simulink model "Copy_2_of_laod_arduino_2021"  (R2020b)
settings: Solver=FixedStepDiscrete  StartTime=0.0  StopTime=Inf  FixedStep=0.02  RelTol=1e-3  EnableMultiTasking=on
values from neighbouring files (symbols this model uses):
  attuatore_Amax = deg2rad(20)    [AVVIO_YAK_DATA.m]
  attuatore_Amin = deg2rad(-20)    [AVVIO_YAK_DATA.m]
  attuatore_Emax = deg2rad(25)    [AVVIO_YAK_DATA.m]
  attuatore_Emin = deg2rad(-25)    [AVVIO_YAK_DATA.m]
  attuatore_Rmax = deg2rad(25)    [AVVIO_YAK_DATA.m]
  attuatore_Rmin = deg2rad(-25)    [AVVIO_YAK_DATA.m]
  attuatore_Tmax = 0.4    [AVVIO_YAK_DATA.m]
  attuatore_Tmin = 0    [AVVIO_YAK_DATA.m]
  interventoA_05 = 6    [AVVIO_YAK_DATA.m]
  interventoA_1 = 2    [AVVIO_YAK_DATA.m]
  interventoE_05 = 7.5    [AVVIO_YAK_DATA.m]
  interventoE_1 = 3.2    [AVVIO_YAK_DATA.m]
  interventoT = 0.1    [AVVIO_YAK_DATA.m]
  inv_A = 1    [AVVIO_YAK_DATA.m]
  inv_comp_h = 1    [AVVIO_YAK_DATA.m]
  inv_E = 1    [AVVIO_YAK_DATA.m]
  inv_R = 1    [AVVIO_YAK_DATA.m]
  inv_T = 1    [AVVIO_YAK_DATA.m]
  K_AW_B_AP_quota = 1000    [AVVIO_YAK_DATA.m]
  K_AW_B_becc = -250    [AVVIO_YAK_DATA.m]
  K_AW_B_imb = 0    [AVVIO_YAK_DATA.m]
  K_AW_B_roll = 500    [AVVIO_YAK_DATA.m]
  K_imb_inv = -1    [AVVIO_YAK_DATA.m]
  Kd_h_app = 0.085    [AVVIO_YAK_DATA.m]
  Kd_h_flare = 0.01    [AVVIO_YAK_DATA.m]
  Ki_AP_quota_select = 0.014    [AVVIO_YAK_DATA.m]
  Ki_AP_rotta = 0.03    [AVVIO_YAK_DATA.m]
  Ki_AP_vel = 0.001    [AVVIO_YAK_DATA.m]
  Ki_becch = -0.064065    [AVVIO_YAK_DATA.m]
  Ki_h_app = 0.055    [AVVIO_YAK_DATA.m]
  Ki_h_cruise = 0.008    [AVVIO_YAK_DATA.m]
  Ki_h_flare = 0.07    [AVVIO_YAK_DATA.m]
  Ki_roll = 0.025    [AVVIO_YAK_DATA.m]
  Kp_AP_quota_hold_h = 0.15    [AVVIO_YAK_DATA.m]
  Kp_AP_quota_hold_l = 0.7    [AVVIO_YAK_DATA.m]
  Kp_AP_quota_select = 0.014    [AVVIO_YAK_DATA.m]
  Kp_AP_rotta = 0.7    [AVVIO_YAK_DATA.m]
  Kp_AP_vel = 0.02692    [AVVIO_YAK_DATA.m]
  Kp_becch = -0.1918    [AVVIO_YAK_DATA.m]
  Kp_comp_h = 0.035    [AVVIO_YAK_DATA.m]
  Kp_h_app_max = 0.086    [AVVIO_YAK_DATA.m]
  Kp_h_app_min = 0.01    [AVVIO_YAK_DATA.m]
  Kp_h_cruise = 0.04    [AVVIO_YAK_DATA.m]
  Kp_h_flare = 0.1    [AVVIO_YAK_DATA.m]
  Kp_imb = -0.04    [AVVIO_YAK_DATA.m]
  Kp_p = 0.025    [AVVIO_YAK_DATA.m]
  Kp_q = -0.025    [AVVIO_YAK_DATA.m]
  Kp_roll = 0.11    [AVVIO_YAK_DATA.m]
  Kp_Rotta_ATO = 4    [AVVIO_YAK_DATA.m]
  safe_phi = 55    [AVVIO_YAK_DATA.m]
  safe_V = 40    [AVVIO_YAK_DATA.m]
  t_AP = 0.02    [AVVIO_YAK_DATA.m]
  time_alarm_SAFE = 1    [AVVIO_YAK_DATA.m]
  V_max = 35    [AVVIO_YAK_DATA.m]
  V_stall = 15    [AVVIO_YAK_DATA.m]
  vel_wp1_al = 25    [AVVIO_YAK_DATA.m]
  vel_wp2_al = 20    [AVVIO_YAK_DATA.m]
undefined symbols (not defined in the file or in its folder): DiscIntNeverNeededParam, Newton, phi_max, phi_min, Raphson, theta_max, theta_min, tsamp
libraries: simulink_extras x43, arduinolib x26, pid_lib x8, svdutilitieslib x6, simulink x3, dspsigops x3, aerolibtransform2sys x2, aerolibtransform2 x2, cstblocks x1
(part 4 of 8)

== system Copy_2_of_laod_arduino_2021/AUTOPILOTA/Subsystem1/DECOLLO AUTOMATICO ==
  Tas : Inport
  h : Inport  Port=2
  modo : Inport  Port=3
  psi_imu : Inport  Port=4
  theta : Inport  Port=5
  V_ : Inport  Port=6
  Enable : EnablePort
  Chart1 : Stateflow chart  TreatAsAtomicUnit=on
  Memory : Memory
  Memory1 : Memory
  Radians to Degrees : simulink_extras/Transformations/Radians to Degrees
  Radians to Degrees1 : simulink_extras/Transformations/Radians to Degrees
  Sample and Hold : dspsigops/Sample and Hold  trig=Rising edge  initCond=0  latchinput=off
  Sample and Hold1 : dspsigops/Sample and Hold  trig=Rising edge  initCond=0  latchinput=off
  rotta_ATO : Outport  VectorParamsAs1DForOutWhenUnconnected=off
  Fase_ATO : Outport  Port=2  VectorParamsAs1DForOutWhenUnconnected=off
  manetta_ref_ATO : Outport  Port=3  VectorParamsAs1DForOutWhenUnconnected=off
  eq_rot_ATO : Outport  Port=4  VectorParamsAs1DForOutWhenUnconnected=off
  phi_ref_ATO : Outport  Port=5  VectorParamsAs1DForOutWhenUnconnected=off
  theta_ref_ATO : Outport  Port=6  VectorParamsAs1DForOutWhenUnconnected=off
  h_ref_ATO : Outport  Port=7  VectorParamsAs1DForOutWhenUnconnected=off
  Tas_ref_ATO : Outport  Port=8  VectorParamsAs1DForOutWhenUnconnected=off
  RC_ref_ATO : Outport  Port=9  VectorParamsAs1DForOutWhenUnconnected=off
  wires:
  Chart1/3(psi_ref) -> rotta_ATO/1  "ROTTA"
  modo/1 -> Chart1/1(modo)
  h/1 -> Chart1/3(h)
  Tas/1 -> Chart1/2(TAS)
  Chart1/10(psi_ref_selector) -> Memory/1
  Memory/1 -> Sample and Hold/Trigger
  Sample and Hold/1 -> Chart1/4(psi_hold)
  psi_imu/1 -> Radians to Degrees1/1
  Chart1/1(Fase_ATO) -> Fase_ATO/1
  Chart1/2(manetta_ref) -> manetta_ref_ATO/1
  Chart1/7(h_ref) -> h_ref_ATO/1
  Chart1/4(eq_rot) -> eq_rot_ATO/1
  Chart1/5(phi_ref) -> phi_ref_ATO/1
  Chart1/6(pitch_ref) -> theta_ref_ATO/1
  Chart1/8(Tas_ref) -> Tas_ref_ATO/1
  Chart1/9(RC_ref) -> RC_ref_ATO/1
  Sample and Hold1/1 -> Chart1/5(theta_ground_hold)
  Chart1/11(theta_ground_selector) -> Memory1/1
  Memory1/1 -> Sample and Hold1/Trigger
  theta/1 -> Radians to Degrees/1
  Radians to Degrees/1 -> Sample and Hold1/1
  V_/1 -> Chart1/6(V_)
  Radians to Degrees1/1 -> Sample and Hold/1

== system Copy_2_of_laod_arduino_2021/AUTOPILOTA/Subsystem1/Subsystem ==
  In1 : Inport
  In2 : Inport  Port=2
  In3 : Inport  Port=3
  In4 : Inport  Port=4
  In5 : Inport  Port=5
  <IAS> : Inport  Port=6
  In7 : Inport  Port=7
  <ALT> : Inport  Port=8
  <HDG> : Inport  Port=9
  In10 : Inport  Port=10
  <RC> : Inport  Port=11
  In12 : Inport  Port=12
  <Ingaggio_AP> : Inport  Port=13
  In14 : Inport  Port=14
  Enable : EnablePort
  Abs : Abs
  Data Type Conversion{,1..3} (4 alike) : DataTypeConversion  OutDataTypeStr=double
  Memory{,1..3,6} (5 alike) : Memory  InheritSampleTime=on
  Radians to Degrees3 : simulink_extras/Transformations/Radians to Degrees
  VETTORIALE : MATLAB Function  TreatAsAtomicUnit=on
  Out1 : Outport  VectorParamsAs1DForOutWhenUnconnected=off
  Out2 : Outport  Port=2  VectorParamsAs1DForOutWhenUnconnected=off
  Out3 : Outport  Port=3  VectorParamsAs1DForOutWhenUnconnected=off
  Out4 : Outport  Port=4  VectorParamsAs1DForOutWhenUnconnected=off
  wires:
  Data Type Conversion1/1 -> VETTORIALE/8(VELOCITA)
  Memory1/1 -> VETTORIALE/18(ALT_pre)
  VETTORIALE/5(ingaggio_AP_mem) -> Memory6/1
  Data Type Conversion2/1 -> VETTORIALE/9(QUOTA)
  VETTORIALE/8(ALT_pre_mem) -> Memory1/1
  Radians to Degrees3/1 -> VETTORIALE/11(HEADING)
  Memory6/1 -> VETTORIALE/15(ingaggio_AP_pre)
  In12/1 -> VETTORIALE/13(h)
  Memory3/1 -> VETTORIALE/16(modo_pre)
  VETTORIALE/6(modo_pre_mem) -> Memory3/1
  Abs/1 -> VETTORIALE/10(RC)
  VETTORIALE/9(HDG_pre_mem) -> Memory/1
  Data Type Conversion3/1 -> Abs/1
  Memory/1 -> VETTORIALE/19(HDG_pre)
  Data Type Conversion/1 -> VETTORIALE/7(ROTTA)
  Memory2/1 -> VETTORIALE/17(IAS_pre)
  VETTORIALE/7(IAS_pre_mem) -> Memory2/1
  VETTORIALE/3(rotta_vett) -> Out3/1
  In1/1 -> VETTORIALE/1(modo)
  <ALT>/1 -> VETTORIALE/3(ALT)
  <RC>/1 -> VETTORIALE/5(I_RC)
  In5/1 -> Data Type Conversion3/1
  In4/1 -> Data Type Conversion2/1
  <Ingaggio_AP>/1 -> VETTORIALE/6(ingaggio_AP)
  In10/1 -> VETTORIALE/12(TAS)
  In7/1 -> Radians to Degrees3/1
  In3/1 -> Data Type Conversion1/1
  VETTORIALE/1(V_vett) -> Out1/1
  VETTORIALE/2(h_vett) -> Out2/1
  <IAS>/1 -> VETTORIALE/2(IAS)
  In2/1 -> Data Type Conversion/1
  In14/1 -> VETTORIALE/14(RC_default)
  VETTORIALE/4(RC_vett) -> Out4/1
  <HDG>/1 -> VETTORIALE/4(HDG)

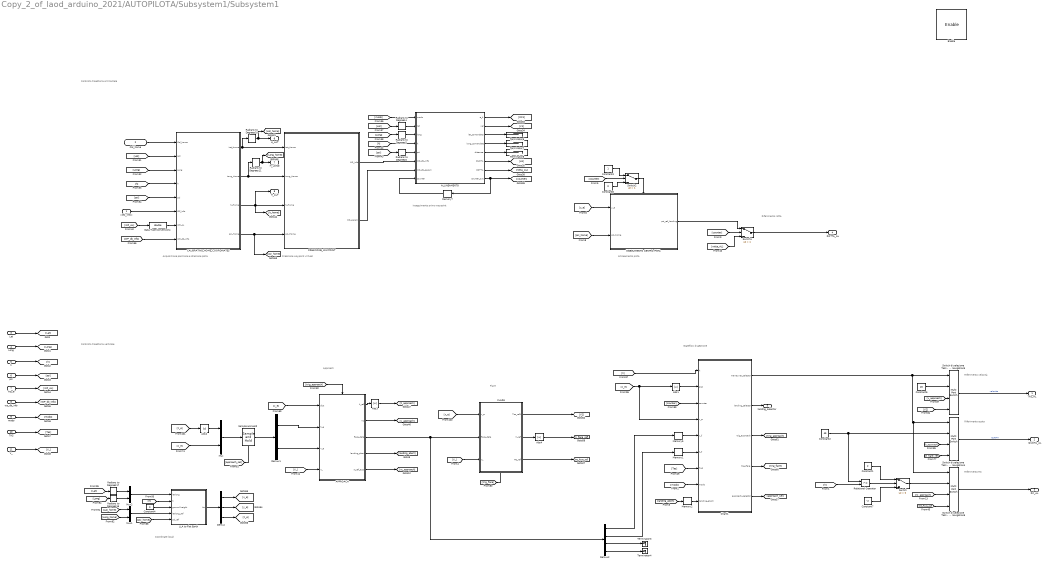
== system Copy_2_of_laod_arduino_2021/AUTOPILOTA/Subsystem1/Subsystem1 ==
  note: Approach
  note: Controllo traiettoria verticale
  note: Flare
  note: Coordinate locali
  note: Stateflow di gestione
  note: Controllo traiettoria orizzontale
  note: Acquisizione posizione
      | e direzione pista
  note: Creazione waypoint
      | virtuali
  note: Inseguimento primo
      | waypoint
  note: Allineamento
      | pista
  note: Riferimento rotta
  note: Riferimento velocità
  note: Riferimento quota
  note: Riferimento RC
  <GC_info> : Inport
  Cal_home : Inport  Port=2
  Lat : Inport  Port=3
  Long : Inport  Port=4
  h : Inport  Port=5
  psi : Inport  Port=6
  wp_al : Inport  Port=7
  wp_db_info : Inport  Port=8
  modo : Inport  Port=9
  TAS : Inport  Port=10
  V_ : Inport  Port=11
  Enable : EnablePort
  ALLINEAMENTO : MATLAB Function  TreatAsAtomicUnit=on
  APPROACH : Subsystem
  Abs{1..4} (4 alike) : Abs
  CALIBRATING_HOME_COORDINATES : MATLAB Function  TreatAsAtomicUnit=on
  "CREAZIONE_WAYPOINT " : Subsystem
  Chart1 : Stateflow chart  TreatAsAtomicUnit=on
  Constant1 : Constant  Value=2  SampleTime=0.02
  Constant2 : Constant  Value=45  SampleTime=0.02
  Constant3 : Constant
  Constant4 : Constant  Value=0  SampleTime=0.02
  Constant6 : Constant  Value=20  SampleTime=0.02
  Constant7 : Constant  Value=-2  SampleTime=0.02
  Constant8 : Constant  Value=0
  Data Type Conversion4 : DataTypeConversion  OutDataTypeStr=double
  Demux : Demux  Outputs=3
  Demux1 : Demux  Outputs=2
  Demux2 : Demux
  FLARE : Subsystem
  INSEGUIMENTO CENTRO PISTA : Subsystem
  LLA to Flat Earth : Subsystem
  Memory1 : Memory
  Memory2 : Memory
  Memory5 : Memory
  Memory7 : Memory  InitialCondition=1  InheritSampleTime=on
  Mux : Mux  Inputs=2
  Mux1 : Mux  Inputs=2
  Mux2 : Mux  Inputs=2
  Radians to Degrees{4..6,10..11,16..17} (7 alike) : simulink_extras/Transformations/Radians to Degrees
  Relational Operator : RelationalOperator  OutDataTypeStr=boolean  RndMeth=Simplest
  Sample and Hold : dspsigops/Sample and Hold  trig=Rising edge  initCond=[0 0]  latchinput=off
  Switch : Switch  Criteria=u2 > Threshold
  Switch di selezione Task - Waypoint navigation4 : MultiPortSwitch
  Switch di selezione Task - Waypoint navigation5 : MultiPortSwitch
  Switch di selezione Task - Waypoint navigation6 : MultiPortSwitch
  Switch1 : Switch  Criteria=u2 > Threshold  Threshold=1
  Switch2 : Switch  Criteria=u2 > Threshold  Threshold=1
  Terminator{3..4,6..8} (5 alike) : Terminator
  TAS_AL : Outport  VectorParamsAs1DForOutWhenUnconnected=off
  QUOTA_AL : Outport  Port=2  VectorParamsAs1DForOutWhenUnconnected=off
  RC_AL : Outport  Port=3  VectorParamsAs1DForOutWhenUnconnected=off
  ROTTA_AL : Outport  Port=4  VectorParamsAs1DForOutWhenUnconnected=off
  landing_selector : Outport  Port=5  VectorParamsAs1DForOutWhenUnconnected=off
  H_LAT : Outport  Port=6  VectorParamsAs1DForOutWhenUnconnected=off
  H_LONG : Outport  Port=7  VectorParamsAs1DForOutWhenUnconnected=off
  H_ALT : Outport  Port=8  VectorParamsAs1DForOutWhenUnconnected=off
  wires:
  Chart1/1(maneuver_selector) -> Switch di selezione Task - Waypoint navigation6/1, Switch di selezione Task - Waypoint navigation4/1, Switch di selezione Task - Waypoint navigation5/1
  LLA to Flat Earth/1(Xe) -> Demux/1
  Radians to Degrees11/1 -> H_LONG/1, [Long_home]
  Mux/1 -> Sample and Hold/1
  ALLINEAMENTO/4(long_comandato) -> Terminator7/1
  Mux1/1 -> LLA to Flat Earth/4(latlong_ref)
  [WP_db_info] -> CALIBRATING_HOME_COORDINATES/8(WP_db_info)
  Demux1/2 -> APPROACH/3(x_g)
  Abs2/1 -> Mux/1
  ALLINEAMENTO/3(lat_comandato) -> Terminator6/1
  [rc_approach] -> Switch di selezione Task - Waypoint navigation6/3
  [V2] -> Switch di selezione Task - Waypoint navigation5/4
  [x_e] -> Chart1/4(x_e), Abs1/1
  Abs4/1 -> [h_flare_ref]
  CALIBRATING_HOME_COORDINATES/3(h_Home) -> H_ALT/1, [h_home], "CREAZIONE_WAYPOINT "/3(h_Home)
  [h] -> Chart1/1(h)
  [x_e] -> FLARE/1(x_e)
  [Long_home] -> Mux1/2
  APPROACH/3(flare_data) -> Demux2/1, FLARE/2(flare_data)
  CALIBRATING_HOME_COORDINATES/1(Lat_Home) -> Radians to Degrees10/1, "CREAZIONE_WAYPOINT "/1(Lat_Home)
  Demux/2 -> [y_e]
  FLARE/3(RC_ref) -> [RC_flare_ref]
  Chart1/4(trig_flare) -> [trig_flare]
  [h] -> LLA to Flat Earth/2(h)
  [Long] -> Radians to Degrees16/1
  Demux/3 -> [z_e]
  Demux2/2 -> Memory1/1
  Radians to Degrees10/1 -> H_LAT/1, [Lat_home]
  Sample and Hold/1 -> Demux1/1
  [trig_approach] -> APPROACH/Enable
  Switch/1 -> Switch di selezione Task - Waypoint navigation6/2
  Memory5/1 -> Chart1/5(x_f)
  Cal_home/1 -> CALIBRATING_HOME_COORDINATES/1(Cal_home)
  Demux2/3 -> Terminator3/1
  FLARE/2(h_ref) -> Abs4/1
  [z_e] -> Abs2/1
  [x_e] -> Mux/2
  CALIBRATING_HOME_COORDINATES/2(Long_Home) -> "CREAZIONE_WAYPOINT "/2(Long_Home), Radians to Degrees11/1
  Demux2/4 -> Terminator4/1
  FLARE/1(Tas_ref1) -> [V2]
  ALLINEAMENTO/7(ROTTA) -> [rotta_AL]
  APPROACH/2(V1) -> [v_approach]
  [V_] -> FLARE/3(V_)
  Chart1/5(approach_selector) -> [approach_sel]
  Abs1/1 -> Chart1/2(dist)
  [h_approach] -> Switch di selezione Task - Waypoint navigation4/3
  [RC_flare_ref] -> Switch di selezione Task - Waypoint navigation6/4
  Chart1/3(trig_approach) -> [trig_approach]
  [Lat_home] -> Mux1/1
  ALLINEAMENTO/6(QUOTA) -> [H1]
  ALLINEAMENTO/8(counter_out) -> Memory7/1, [counter]
  Demux/1 -> [x_e]
  Demux2/1 -> Memory5/1
  CALIBRATING_HOME_COORDINATES/4(psi_Home) -> [psi_home], "CREAZIONE_WAYPOINT "/4(psi_Home)
  Abs3/1 -> [h_approach]
  Mux2/1 -> LLA to Flat Earth/1(latlong)
  Chart1/2(landing_selector) -> landing_selector/1
  Constant2/1 -> Switch di selezione Task - Waypoint navigation4/2, Relational Operator/1
  [h_flare_ref] -> Switch di selezione Task - Waypoint navigation4/4
  [v_approach] -> Switch di selezione Task - Waypoint navigation5/3
  [Tas] -> Chart1/7(TAS)
  APPROACH/1(h_ref) -> Abs3/1
  Data Type Conversion4/1 -> CALIBRATING_HOME_COORDINATES/7(WP_AL)
  [Lat] -> Radians to Degrees17/1
  Demux1/1 -> APPROACH/2(h_g)
  Constant4/1 -> LLA to Flat Earth/3(ground height)
  [psi] -> CALIBRATING_HOME_COORDINATES/5(psi)
  ALLINEAMENTO/2(vel) -> [V1]
  Radians to Degrees5/1 -> ALLINEAMENTO/3(long)
  [x_e] -> APPROACH/1(dist)
  Memory7/1 -> ALLINEAMENTO/8(counter)
  [h] -> CALIBRATING_HOME_COORDINATES/4(h)
  [counter] -> Chart1/3(counter)
  Radians to Degrees4/1 -> ALLINEAMENTO/2(lat)
  [approach_sel] -> Sample and Hold/Trigger
  [Lat] -> Radians to Degrees4/1
  "CREAZIONE_WAYPOINT "/2(WP_param) -> ALLINEAMENTO/7(WP_db_param)
  [h] -> ALLINEAMENTO/4(h)
  [Long] -> Radians to Degrees5/1
  <GC_info>/1 -> CALIBRATING_HOME_COORDINATES/6(GC_info)
  ALLINEAMENTO/1(e_h) -> [RC1]
  Radians to Degrees6/1 -> ALLINEAMENTO/5(psi)
  Radians to Degrees16/1 -> Mux2/2
  [psi] -> Radians to Degrees6/1
  [WP_AL] -> Data Type Conversion4/1
  [modo] -> ALLINEAMENTO/1(modo)
  ALLINEAMENTO/5(distance) -> Terminator8/1
  Radians to Degrees17/1 -> Mux2/1
  "CREAZIONE_WAYPOINT "/1(WP_info) -> ALLINEAMENTO/6(WP_db_info)
  [trig_flare] -> FLARE/Enable
  Constant6/1 -> Switch di selezione Task - Waypoint navigation5/2
  [psi_home] -> LLA to Flat Earth/5(psi_ref)
  Switch di selezione Task - Waypoint navigation4/1 -> QUOTA_AL/1  "QUOTA"
  Switch di selezione Task - Waypoint navigation6/1 -> RC_AL/1
  Switch di selezione Task - Waypoint navigation5/1 -> TAS_AL/1  "velocita"
  Lat/1 -> [Lat]
  Long/1 -> [Long]
  h/1 -> [h]
  psi/1 -> [psi]
  wp_al/1 -> [WP_AL]
  wp_db_info/1 -> [WP_db_info]
  modo/1 -> [modo]
  TAS/1 -> [Tas]
  V_/1 -> [V_]
  Switch1/1 -> ROTTA_AL/1
  [h] -> Relational Operator/2
  Relational Operator/1 -> Switch/2
  Constant1/1 -> Switch/1
  Constant7/1 -> Switch/3
  [modo] -> Chart1/8(modo)
  APPROACH/4(landing_abort) -> [landing_abort]
  Memory1/1 -> Chart1/6(h_f)
  Memory2/1 -> Chart1/9(landing_abort)
  [landing_abort] -> Memory2/1
  [Lat] -> CALIBRATING_HOME_COORDINATES/2(Lat)
  [Long] -> CALIBRATING_HOME_COORDINATES/3(Long)
  [counter] -> Switch2/2
  [rotta_AL] -> Switch1/3
  [psi_home] -> INSEGUIMENTO CENTRO PISTA/2(psi_home)
  INSEGUIMENTO CENTRO PISTA/1(psi_ref_landing) -> Switch1/1
  [y_e] -> INSEGUIMENTO CENTRO PISTA/1(y_e)
  [counter] -> Switch1/2
  Constant8/1 -> Switch2/3
  Switch2/1 -> INSEGUIMENTO CENTRO PISTA/Enable
  Constant3/1 -> Switch2/1
  [V_] -> APPROACH/4(V_)
  APPROACH/5(rc_ref_app) -> [rc_approach]

== system Copy_2_of_laod_arduino_2021/AUTOPILOTA/Subsystem1/Subsystem2 ==
  In1 : Inport
  In2 : Inport  Port=2
  In3 : Inport  Port=3
  In4 : Inport  Port=4
  In5 : Inport  Port=5
  In6 : Inport  Port=6
  <GC_info> : Inport  Port=7
  Enable : EnablePort
  Memory4 : Memory  InitialCondition=1  InheritSampleTime=on
  Radians to Degrees : simulink_extras/Transformations/Radians to Degrees
  Radians to Degrees1 : simulink_extras/Transformations/Radians to Degrees
  Radians to Degrees2 : simulink_extras/Transformations/Radians to Degrees
  Terminator : Terminator
  Terminator1 : Terminator
  Terminator2 : Terminator
  WAYPOINTS : MATLAB Function  TreatAsAtomicUnit=on
  saturatore V : Saturate  UpperLimit=40  LowerLimit=15
  saturatore V1 : Saturate  UpperLimit=2  LowerLimit=-2
  RC : Outport  VectorParamsAs1DForOutWhenUnconnected=off
  VELOCITA : Outport  Port=2  VectorParamsAs1DForOutWhenUnconnected=off
  Out3 : Outport  Port=3  VectorParamsAs1DForOutWhenUnconnected=off
  Out4 : Outport  Port=4  VectorParamsAs1DForOutWhenUnconnected=off
  wires:
  WAYPOINTS/8(counter_out) -> Memory4/1
  saturatore V1/1 -> RC/1  "RC"
  Radians to Degrees1/1 -> WAYPOINTS/2(long)
  WAYPOINTS/4(long_comandato) -> Terminator1/1
  Radians to Degrees/1 -> WAYPOINTS/1(lat)
  WAYPOINTS/2(vel) -> saturatore V/1
  WAYPOINTS/1(e_h) -> saturatore V1/1
  WAYPOINTS/5(distance) -> Terminator2/1
  WAYPOINTS/3(lat_comandato) -> Terminator/1
  Radians to Degrees2/1 -> WAYPOINTS/4(psi)
  Memory4/1 -> WAYPOINTS/8(counter)
  In1/1 -> Radians to Degrees/1
  In3/1 -> WAYPOINTS/3(h)
  In4/1 -> Radians to Degrees2/1
  In2/1 -> Radians to Degrees1/1
  WAYPOINTS/7(ROTTA) -> Out4/1
  In5/1 -> WAYPOINTS/5(WP_db_info)
  In6/1 -> WAYPOINTS/6(WP_db_param)
  <GC_info>/1 -> WAYPOINTS/7(GC_info)
  saturatore V/1 -> VELOCITA/1  "VELOCITA"
  WAYPOINTS/6(QUOTA) -> Out3/1

== system Copy_2_of_laod_arduino_2021/AUTOPILOTA/Subsystem1/Subsystem3 ==
  In1 : Inport
  In2 : Inport  Port=2
  In3 : Inport  Port=3
  In4 : Inport  Port=4
  In5 : Inport  Port=5
  In6 : Inport  Port=6
  In7 : Inport  Port=7
  In8 : Inport  Port=8
  Enable : EnablePort
  GO_HOME : MATLAB Function  TreatAsAtomicUnit=on
  Radians to Degrees12 : simulink_extras/Transformations/Radians to Degrees
  Radians to Degrees13 : simulink_extras/Transformations/Radians to Degrees
  Radians to Degrees9 : simulink_extras/Transformations/Radians to Degrees
  Out1 : Outport  VectorParamsAs1DForOutWhenUnconnected=off
  Out2 : Outport  Port=2  VectorParamsAs1DForOutWhenUnconnected=off
  Out3 : Outport  Port=3  VectorParamsAs1DForOutWhenUnconnected=off
  Out4 : Outport  Port=4  VectorParamsAs1DForOutWhenUnconnected=off
  wires:
  GO_HOME/1(V_goHome) -> Out1/1
  GO_HOME/4(rotta_goHome) -> Out4/1
  GO_HOME/3(RC_goHome) -> Out3/1
  Radians to Degrees9/1 -> GO_HOME/4(psi)
  Radians to Degrees12/1 -> GO_HOME/1(lat)
  In2/1 -> Radians to Degrees13/1
  Radians to Degrees13/1 -> GO_HOME/2(long)
  In3/1 -> GO_HOME/3(h)
  In4/1 -> Radians to Degrees9/1
  In6/1 -> GO_HOME/6(Long_Home)
  In8/1 -> GO_HOME/8(V_goHome_rif)
  In5/1 -> GO_HOME/5(Lat_Home)
  In1/1 -> Radians to Degrees12/1
  GO_HOME/2(h_goHome) -> Out2/1
  In7/1 -> GO_HOME/7(h_goHome_rif)

== system Copy_2_of_laod_arduino_2021/MISURE DA SENSORI FILTRATE/TX & RX Seriale Arduino Raspberry/Subsystem1 ==
  In1 : Inport
  Enable : EnablePort
  MATLAB Function : MATLAB Function  TreatAsAtomicUnit=on
  MATLAB Function1 : MATLAB Function  Commented=on  TreatAsAtomicUnit=on
  Subsystem1 : Subsystem  Commented=on
  Subsystem2 : Subsystem
  Terminator : Terminator  Commented=on
  Transpose : Math  Operator=transpose  SignedPower=on  SaturateOnIntegerOverflow=on
  Unit Delay : UnitDelay  Commented=on  SampleTime=-1  HasFrameUpgradeWarning=on
  Single : Outport  VectorParamsAs1DForOutWhenUnconnected=off
  Int16 : Outport  Port=2  VectorParamsAs1DForOutWhenUnconnected=off
  uint16 : Outport  Port=3  VectorParamsAs1DForOutWhenUnconnected=off
  wires:
  In1/1 -> Transpose/1
  Subsystem2/1(Out2) -> Single/1
  Subsystem2/2(Out3) -> Int16/1
  Subsystem2/3(Out4) -> uint16/1
  MATLAB Function/1(status) -> Subsystem2/Enable
  MATLAB Function/2(messaggio) -> Subsystem2/1(In1)
  MATLAB Function1/1(status) -> Subsystem1/Enable
  MATLAB Function1/3(messaggio) -> Subsystem1/1(In1), Unit Delay/1
  Unit Delay/1 -> MATLAB Function1/2(mess_prec)
  MATLAB Function1/2(check) -> Terminator/1
  Transpose/1 -> MATLAB Function/1(byte_pack)

== system Copy_2_of_laod_arduino_2021/Misure Sensori/ATTOPILOT/Scalatura_bit_to_percent_Volt ==
  Bit : Inport
  Sum : Sum  Inputs=|++
  m_attopilota_bit_to_percent : Gain  Gain=100/361  ParamDataTypeStr=double
  q_attopilota_bit_to_percent : Constant  Value=-204800/361
  Percent_Volt : Outport  VectorParamsAs1DForOutWhenUnconnected=off
  wires:
  Bit/1 -> m_attopilota_bit_to_percent/1
  Sum/1 -> Percent_Volt/1
  q_attopilota_bit_to_percent/1 -> Sum/2
  m_attopilota_bit_to_percent/1 -> Sum/1

== system Copy_2_of_laod_arduino_2021/Misure Sensori/BMP_280/Dynamic rate limiter ==
  note: U(k)
  note: Y(k)
  up : Inport
  u : Inport  Port=2
  lo : Inport  Port=3
  Delay Input2 : UnitDelay  Description=Store in Global RAM  DisableCoverage=on  InitialCondition=101325  SampleTime=-1  HasFrameUpgradeWarning=on
  Difference Inputs1 : Sum  Description=Add in CPU  DisableCoverage=on  Inputs=+-  OutDataTypeStr=Inherit: Inherit via back propagation
  Difference Inputs2 : Sum  Description=Add in CPU  OutDataTypeStr=Inherit: Inherit via back propagation
  FixPt Data Type Duplicate : DataTypeDuplicate  DisableCoverage=on  NumInputPorts=7
  Saturation Dynamic : simulink/Discontinuities/Saturation Dynamic  OutMin=[]  OutMax=[]  OutDataTypeStr=Inherit: Same as second input  OutDataType=fixdt(1, 16)  OutScaling=2^-10  DoSatur=off
  delta fall limit : Product  DisableCoverage=on  Inputs=**  OutDataTypeStr=Inherit: Inherit via back propagation  SaturateOnIntegerOverflow=on
  delta rise limit : Product  DisableCoverage=on  Inputs=**  OutDataTypeStr=Inherit: Inherit via back propagation  SaturateOnIntegerOverflow=on
  sample time : SampleTimeMath  DisableCoverage=on  TsampMathOp=Ts Only  weightValue=1
  Y : Outport  InitialOutput=0  VectorParamsAs1DForOutWhenUnconnected=off
  wires:
  delta rise limit/1 -> FixPt Data Type Duplicate/6, Saturation Dynamic/1
  Difference Inputs2/1 -> Y/1, Delay Input2/1, FixPt Data Type Duplicate/1
  up/1 -> delta rise limit/1
  Saturation Dynamic/1 -> Difference Inputs2/1, FixPt Data Type Duplicate/7
  Delay Input2/1 -> Difference Inputs1/2, FixPt Data Type Duplicate/2, Difference Inputs2/2  "Y(k-1)"
  Difference Inputs1/1 -> FixPt Data Type Duplicate/4, Saturation Dynamic/2  "( U(k) - Y(k-1) )"
  u/1 -> Difference Inputs1/1, FixPt Data Type Duplicate/5, sample time/1
  lo/1 -> delta fall limit/1
  sample time/1 -> delta fall limit/2, delta rise limit/2
  delta fall limit/1 -> FixPt Data Type Duplicate/3, Saturation Dynamic/3

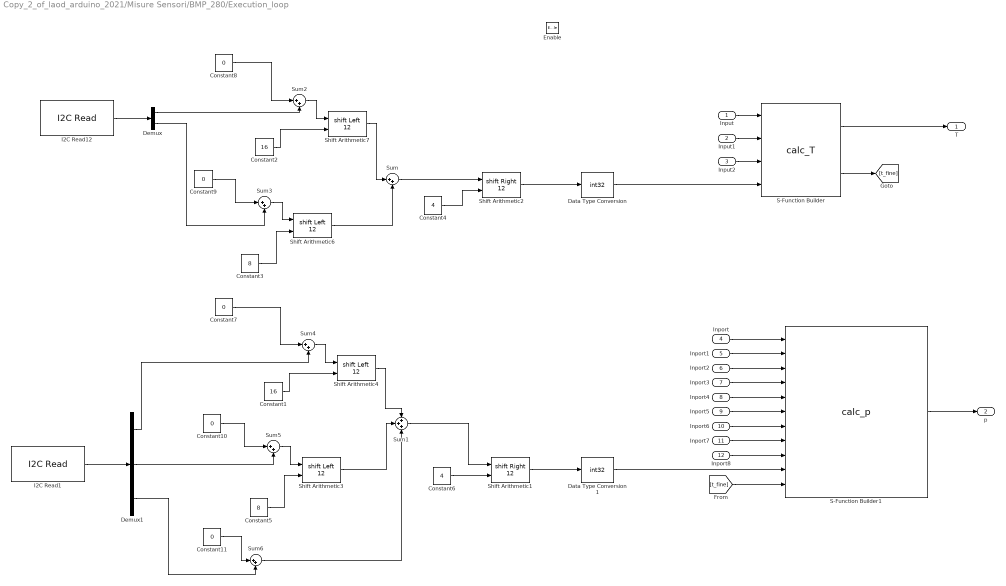
== system Copy_2_of_laod_arduino_2021/Misure Sensori/BMP_280/Execution_loop ==
  Input : Inport
  Input1 : Inport  Port=2
  Input2 : Inport  Port=3
  Inport : Inport  Port=4
  Inport1 : Inport  Port=5
  Inport2 : Inport  Port=6
  Inport3 : Inport  Port=7
  Inport4 : Inport  Port=8
  Inport5 : Inport  Port=9
  Inport6 : Inport  Port=10
  Inport7 : Inport  Port=11
  Inport8 : Inport  Port=12
  Enable : EnablePort
  Constant1 : Constant  Value=16
  Constant{7..11} (5 alike) : Constant  Value=0  OutDataTypeStr=uint32
  Constant2 : Constant  Value=16
  Constant3 : Constant  Value=8
  Constant4 : Constant  Value=4
  Constant5 : Constant  Value=8
  Constant6 : Constant  Value=4
  Data Type Conversion : DataTypeConversion  OutDataTypeStr=int32
  Data Type Conversion1 : DataTypeConversion  OutDataTypeStr=int32
  Demux : Demux  Outputs=2
  Demux1 : Demux  Outputs=3
  I2C Read1 : arduinolib/I2C Read  Priority=2  I2CModule=0  Mode=Master  SlaveAddress=hex2dec( '76' )  SlaveByteOrder=BigEndian  Direction=Receiver  RegisterAddressMode=on  RegisterAddress=hex2dec( 'F7' )  SlaveDataType=uint8  DataLength=3  NoAck=off  RepeatedStart=off  OutputStatus=off  blockPlatform=arduino  SampleTime=t_AP
      settings: AttributesFormatString=Priority=%<Priority>  SourceProductBaseCode=ARDUINO
  I2C Read12 : arduinolib/I2C Read  Priority=1  I2CModule=0  Mode=Master  SlaveAddress=hex2dec( '76' )  SlaveByteOrder=BigEndian  Direction=Receiver  RegisterAddressMode=on  RegisterAddress=hex2dec( 'FA' )  SlaveDataType=uint8  DataLength=2  NoAck=off  RepeatedStart=off  OutputStatus=off  blockPlatform=arduino  SampleTime=t_AP
      settings: AttributesFormatString=Priority=%<Priority>  SourceProductBaseCode=ARDUINO
  S-Function Builder : S-Function  InitFcn=try, set_param(gcb,'FunctionName','calc_T'), end  FunctionName=calc_T  SFunctionModules=calc_T_wrapper  SFunctionDeploymentMode=off  EnableBusSupport=off  mask(S-Function Builder){}
      mask help: Simulink:masks:SFunctionBuilder_MD
      mask init: same as Copy_2_of_laod_arduino_2021/AIR RX/S-Function Builder
      settings: CopyFcn=set_param(gcbh,'LinkStatus','none')  PreSaveFcn=try, set_param(gcb,'FunctionName','calc_T'), end  OpenFcn=sfunctionwizard(gcbh)
      mask Display: plot(val(:,1),val(:,2)),disp(sys), port_label('input',1,'dig_T1'), port_label('input',2,'dig_T2'), port_label('input',3,'dig_T3'), port_label('input',4,'adc_T'), port_label('output',1,'T'), port_label('output',2,'t_fine')
  S-Function Builder1 : S-Function  InitFcn=try, set_param(gcb,'FunctionName','calc_p'), end  FunctionName=calc_p  SFunctionModules=calc_p_wrapper  SFunctionDeploymentMode=off  EnableBusSupport=off  mask(S-Function Builder){}
      mask help: Simulink:masks:SFunctionBuilder_MD
      mask init: same as Copy_2_of_laod_arduino_2021/AIR RX/S-Function Builder
      settings: CopyFcn=set_param(gcbh,'LinkStatus','none')  PreSaveFcn=try, set_param(gcb,'FunctionName','calc_p'), end  OpenFcn=sfunctionwizard(gcbh)
      mask Display: plot(val(:,1),val(:,2)),disp(sys), port_label('input',1,'dig_p1'), port_label('input',2,'dig_p2'), port_label('input',3,'dig_p3'), port_label('input',4,'dig_p4'), port_label('input',5,'dig_p5'), port_label('input',6,'dig_p6'), port_label('input',7,'dig_p7'), port_label('input',8,'dig_p8'), port_label('input',9,'dig_p9'), port_label('input',10,'adc_P'), port_label('input',11,'t_fine'), port_label('output',1,'p')
  Shift Arithmetic1 : ArithShift  BitShiftNumberSource=Input port  BitShiftNumber=12  BitShiftDirection=Right
      settings: InputPortMap=u0,p1
  Shift Arithmetic2 : ArithShift  BitShiftNumberSource=Input port  BitShiftNumber=12  BitShiftDirection=Right
      settings: InputPortMap=u0,p1
  Shift Arithmetic{3..4,6..7} (4 alike) : ArithShift  BitShiftNumberSource=Input port  BitShiftNumber=12  BitShiftDirection=Left
      settings: InputPortMap=u0,p1
  Sum{,2..6} (6 alike) : Sum  Inputs=|++
  Sum1 : Sum  Inputs=+++
  T : Outport  VectorParamsAs1DForOutWhenUnconnected=off
  p : Outport  Port=2  VectorParamsAs1DForOutWhenUnconnected=off
  wires:
  Shift Arithmetic2/1 -> Data Type Conversion/1
  Constant4/1 -> Shift Arithmetic2/2
  S-Function Builder/1 -> T/1
  Input2/1 -> S-Function Builder/3
  Input1/1 -> S-Function Builder/2
  Input/1 -> S-Function Builder/1
  Constant3/1 -> Shift Arithmetic6/2
  Constant2/1 -> Shift Arithmetic7/2
  Shift Arithmetic7/1 -> Sum/1
  Shift Arithmetic6/1 -> Sum/2
  Sum/1 -> Shift Arithmetic2/1
  Sum2/1 -> Shift Arithmetic7/1
  Constant8/1 -> Sum2/1
  Constant9/1 -> Sum3/1
  Demux/2 -> Sum3/2
  Sum3/1 -> Shift Arithmetic6/1
  Data Type Conversion/1 -> S-Function Builder/4
  Shift Arithmetic4/1 -> Sum1/1
  Constant5/1 -> Shift Arithmetic3/2
  Shift Arithmetic1/1 -> Data Type Conversion1/1
  Constant1/1 -> Shift Arithmetic4/2
  Constant6/1 -> Shift Arithmetic1/2
  Sum1/1 -> Shift Arithmetic1/1
  Constant7/1 -> Sum4/1
  S-Function Builder1/1 -> p/1
  Sum5/1 -> Shift Arithmetic3/1
  Constant10/1 -> Sum5/1
  Demux1/2 -> Sum5/2
  Shift Arithmetic3/1 -> Sum1/2
  Sum4/1 -> Shift Arithmetic4/1
  Constant11/1 -> Sum6/1
  Demux1/3 -> Sum6/2
  Sum6/1 -> Sum1/3
  Data Type Conversion1/1 -> S-Function Builder1/10
  Inport/1 -> S-Function Builder1/1
  Inport1/1 -> S-Function Builder1/2
  Inport2/1 -> S-Function Builder1/3
  Inport3/1 -> S-Function Builder1/4
  Inport4/1 -> S-Function Builder1/5
  Inport5/1 -> S-Function Builder1/6
  Inport6/1 -> S-Function Builder1/7
  Inport7/1 -> S-Function Builder1/8
  Inport8/1 -> S-Function Builder1/9
  S-Function Builder/2 -> [t_fine]
  [t_fine] -> S-Function Builder1/11
  I2C Read12/1 -> Demux/1
  Demux/1 -> Sum2/2
  I2C Read1/1 -> Demux1/1
  Demux1/1 -> Sum4/2

== system Copy_2_of_laod_arduino_2021/Misure Sensori/BMP_280/One_time_initialization ==
  Enable : EnablePort
  Bitwise Operator1 : simulink/Logic and Bit Operations/Bitwise Operator  logicop=AND  UseBitMask=on  BitMask=hex2dec('FF')  BitMaskRealWorld=Stored Integer
  Byte Unpack : svdutilitieslib/Byte Unpack  dimensions={[8]}  datatypes={'uint16'}  byteAlign=1  blockPlatform=arduinoert
      settings: SourceProductBaseCode=ANDROID,ARDUINO,ML_ARDUINO,ECCORTEXA,ECCORTEXR,SC_BEAGLEBONE_BLUE,EC_FREEDOM_BOARD,EC_FRDM_K64F,INTEL_BLOCKSET,JETSONCPU,MICROBIT,NUCLEO,NVIDIA,PX4AUTOPILOTS,RASPPIIO,STMICRODIS,TIC2000,XILINX_BLOCKSET
  Constant1 : Constant  Value=hex2dec('0')  OutDataTypeStr=uint8  SampleTime=-1
  Constant4 : Constant  Value=hex2dec('2F')  OutDataTypeStr=uint8  SampleTime=-1
  Data Type Conversion10 : DataTypeConversion  OutDataTypeStr=uint8
  Data Type Conversion11 : DataTypeConversion  OutDataTypeStr=uint8
  I2C Read : arduinolib/I2C Read  Priority=1  I2CModule=0  Mode=Master  SlaveAddress=hex2dec( '76' )  SlaveByteOrder=LittleEndian  Direction=Receiver  RegisterAddressMode=on  RegisterAddress=hex2dec( '88' )  SlaveDataType=uint16  DataLength=1  NoAck=off  RepeatedStart=off  OutputStatus=off  blockPlatform=arduino  SampleTime=t_AP
      settings: AttributesFormatString=Priority=%<Priority>  SourceProductBaseCode=ARDUINO
  I2C Read1 : arduinolib/I2C Read  Priority=2  I2CModule=0  Mode=Master  SlaveAddress=hex2dec( '76' )  SlaveByteOrder=LittleEndian  Direction=Receiver  RegisterAddressMode=on  RegisterAddress=hex2dec( '8A' )  SlaveDataType=int16  DataLength=1  NoAck=off  RepeatedStart=off  OutputStatus=off  blockPlatform=arduino  SampleTime=t_AP
      settings: AttributesFormatString=Priority=%<Priority>  SourceProductBaseCode=ARDUINO
  I2C Read10 : arduinolib/I2C Read  Priority=11  I2CModule=0  Mode=Master  SlaveAddress=hex2dec( '76' )  SlaveByteOrder=LittleEndian  Direction=Receiver  RegisterAddressMode=on  RegisterAddress=hex2dec( '9C' )  SlaveDataType=int16  DataLength=1  NoAck=off  RepeatedStart=off  OutputStatus=off  blockPlatform=arduino  SampleTime=t_AP
      settings: AttributesFormatString=Priority=%<Priority>  SourceProductBaseCode=ARDUINO
  I2C Read11 : arduinolib/I2C Read  Priority=12  I2CModule=0  Mode=Master  SlaveAddress=hex2dec( '76' )  SlaveByteOrder=LittleEndian  Direction=Receiver  RegisterAddressMode=on  RegisterAddress=hex2dec( '9E' )  SlaveDataType=int16  DataLength=1  NoAck=off  RepeatedStart=off  OutputStatus=off  blockPlatform=arduino  SampleTime=t_AP
      settings: AttributesFormatString=Priority=%<Priority>  SourceProductBaseCode=ARDUINO
  I2C Read12 : arduinolib/I2C Read  Priority=16  I2CModule=0  Mode=Master  SlaveAddress=hex2dec( '50' )  SlaveByteOrder=BigEndian  Direction=Receiver  RegisterAddressMode=off  RegisterAddress=0  SlaveDataType=uint8  DataLength=16  NoAck=off  RepeatedStart=off  OutputStatus=off  blockPlatform=ARDUINO  SampleTime=0.02
      settings: AttributesFormatString=Priority=%<Priority>  SourceProductBaseCode=ARDUINO
  I2C Read2 : arduinolib/I2C Read  Priority=3  I2CModule=0  Mode=Master  SlaveAddress=hex2dec( '76' )  SlaveByteOrder=LittleEndian  Direction=Receiver  RegisterAddressMode=on  RegisterAddress=hex2dec( '8C' )  SlaveDataType=int16  DataLength=1  NoAck=off  RepeatedStart=off  OutputStatus=off  blockPlatform=arduino  SampleTime=t_AP
      settings: AttributesFormatString=Priority=%<Priority>  SourceProductBaseCode=ARDUINO
  I2C Read3 : arduinolib/I2C Read  Priority=4  I2CModule=0  Mode=Master  SlaveAddress=hex2dec( '76' )  SlaveByteOrder=LittleEndian  Direction=Receiver  RegisterAddressMode=on  RegisterAddress=hex2dec( '8E' )  SlaveDataType=uint16  DataLength=1  NoAck=off  RepeatedStart=off  OutputStatus=off  blockPlatform=arduino  SampleTime=t_AP
      settings: AttributesFormatString=Priority=%<Priority>  SourceProductBaseCode=ARDUINO
  I2C Read4 : arduinolib/I2C Read  Priority=5  I2CModule=0  Mode=Master  SlaveAddress=hex2dec( '76' )  SlaveByteOrder=LittleEndian  Direction=Receiver  RegisterAddressMode=on  RegisterAddress=hex2dec( '90' )  SlaveDataType=int16  DataLength=1  NoAck=off  RepeatedStart=off  OutputStatus=off  blockPlatform=arduino  SampleTime=t_AP
      settings: AttributesFormatString=Priority=%<Priority>  SourceProductBaseCode=ARDUINO
  I2C Read5 : arduinolib/I2C Read  Priority=6  I2CModule=0  Mode=Master  SlaveAddress=hex2dec( '76' )  SlaveByteOrder=LittleEndian  Direction=Receiver  RegisterAddressMode=on  RegisterAddress=hex2dec( '92' )  SlaveDataType=int16  DataLength=1  NoAck=off  RepeatedStart=off  OutputStatus=off  blockPlatform=arduino  SampleTime=t_AP
      settings: AttributesFormatString=Priority=%<Priority>  SourceProductBaseCode=ARDUINO
  I2C Read6 : arduinolib/I2C Read  Priority=7  I2CModule=0  Mode=Master  SlaveAddress=hex2dec( '76' )  SlaveByteOrder=LittleEndian  Direction=Receiver  RegisterAddressMode=on  RegisterAddress=hex2dec( '94' )  SlaveDataType=int16  DataLength=1  NoAck=off  RepeatedStart=off  OutputStatus=off  blockPlatform=arduino  SampleTime=t_AP
      settings: AttributesFormatString=Priority=%<Priority>  SourceProductBaseCode=ARDUINO
  I2C Read7 : arduinolib/I2C Read  Priority=8  I2CModule=0  Mode=Master  SlaveAddress=hex2dec( '76' )  SlaveByteOrder=LittleEndian  Direction=Receiver  RegisterAddressMode=on  RegisterAddress=hex2dec( '96' )  SlaveDataType=int16  DataLength=1  NoAck=off  RepeatedStart=off  OutputStatus=off  blockPlatform=arduino  SampleTime=t_AP
      settings: AttributesFormatString=Priority=%<Priority>  SourceProductBaseCode=ARDUINO
  I2C Read8 : arduinolib/I2C Read  Priority=9  I2CModule=0  Mode=Master  SlaveAddress=hex2dec( '76' )  SlaveByteOrder=LittleEndian  Direction=Receiver  RegisterAddressMode=on  RegisterAddress=hex2dec( '98' )  SlaveDataType=int16  DataLength=1  NoAck=off  RepeatedStart=off  OutputStatus=off  blockPlatform=arduino  SampleTime=t_AP
      settings: AttributesFormatString=Priority=%<Priority>  SourceProductBaseCode=ARDUINO
  I2C Read9 : arduinolib/I2C Read  Priority=10  I2CModule=0  Mode=Master  SlaveAddress=hex2dec( '76' )  SlaveByteOrder=LittleEndian  Direction=Receiver  RegisterAddressMode=on  RegisterAddress=hex2dec( '9A' )  SlaveDataType=int16  DataLength=1  NoAck=off  RepeatedStart=off  OutputStatus=off  blockPlatform=arduino  SampleTime=t_AP
      settings: AttributesFormatString=Priority=%<Priority>  SourceProductBaseCode=ARDUINO
  I2C Write1 : arduinolib/I2C Write  Priority=13  I2CModule=0  Mode=Master  SlaveAddress=hex2dec( '76' )  SlaveByteOrder=LittleEndian  Direction=Transmitter  RegisterAddressMode=on  RegisterAddress=hex2dec( 'F4' )  SlaveDataType=uint8  DataLength=1  NoAck=off  RepeatedStart=off  OutputStatus=off  blockPlatform=arduino
      settings: AttributesFormatString=Priority=%<Priority>  SourceProductBaseCode=ARDUINO
  I2C Write2 : arduinolib/I2C Write  Priority=14  I2CModule=0  Mode=Master  SlaveAddress=hex2dec( '76' )  SlaveByteOrder=LittleEndian  Direction=Transmitter  RegisterAddressMode=on  RegisterAddress=hex2dec( 'F5' )  SlaveDataType=uint8  DataLength=1  NoAck=off  RepeatedStart=off  OutputStatus=off  blockPlatform=arduino
      settings: AttributesFormatString=Priority=%<Priority>  SourceProductBaseCode=ARDUINO
  I2C Write3 : arduinolib/I2C Write  Priority=15  I2CModule=0  Mode=Master  SlaveAddress=hex2dec( '50' )  SlaveByteOrder=BigEndian  Direction=Transmitter  RegisterAddressMode=off  RegisterAddress=hex2dec( '0' )  SlaveDataType=uint8  DataLength=1  NoAck=off  RepeatedStart=off  OutputStatus=off  blockPlatform=ARDUINO
      settings: AttributesFormatString=Priority=%<Priority>  SourceProductBaseCode=ARDUINO
  Mux1 : Mux  Inputs=2
  Shift Arithmetic1 : ArithShift  BitShiftNumber=8  BitShiftDirection=Right
  "registro memoria2 " : Constant  Value=0  OutDataTypeStr=uint16  SampleTime=t_AP
  dig_T1 : Outport  VectorParamsAs1DForOutWhenUnconnected=off
  dig_T2 : Outport  Port=2  VectorParamsAs1DForOutWhenUnconnected=off
  dig_T3 : Outport  Port=3  VectorParamsAs1DForOutWhenUnconnected=off
  dig_p1 : Outport  Port=4  VectorParamsAs1DForOutWhenUnconnected=off
  dig_p2 : Outport  Port=5  VectorParamsAs1DForOutWhenUnconnected=off
  dig_p3 : Outport  Port=6  VectorParamsAs1DForOutWhenUnconnected=off
  dig_p4 : Outport  Port=7  VectorParamsAs1DForOutWhenUnconnected=off
  dig_p5 : Outport  Port=8  VectorParamsAs1DForOutWhenUnconnected=off
  dig_p6 : Outport  Port=9  VectorParamsAs1DForOutWhenUnconnected=off
  dig_p7 : Outport  Port=10  VectorParamsAs1DForOutWhenUnconnected=off
  dig_p8 : Outport  Port=11  VectorParamsAs1DForOutWhenUnconnected=off
  dig_p9 : Outport  Port=12  VectorParamsAs1DForOutWhenUnconnected=off
  pwm_max_min : Outport  Port=13  VectorParamsAs1DForOutWhenUnconnected=off
  wires:
  Byte Unpack/1 -> pwm_max_min/1
  Data Type Conversion11/1 -> Mux1/2
  "registro memoria2 "/1 -> Bitwise Operator1/1, Shift Arithmetic1/1
  Bitwise Operator1/1 -> Data Type Conversion11/1
  Mux1/1 -> I2C Write3/1
  Shift Arithmetic1/1 -> Data Type Conversion10/1
  Data Type Conversion10/1 -> Mux1/1
  I2C Read12/1 -> Byte Unpack/1
  Constant1/1 -> I2C Write2/1
  Constant4/1 -> I2C Write1/1
  I2C Read1/1 -> dig_T2/1
  I2C Read3/1 -> dig_p1/1
  I2C Read11/1 -> dig_p9/1
  I2C Read9/1 -> dig_p7/1
  I2C Read2/1 -> dig_T3/1
  I2C Read6/1 -> dig_p4/1
  I2C Read5/1 -> dig_p3/1
  I2C Read/1 -> dig_T1/1
  I2C Read4/1 -> dig_p2/1
  I2C Read10/1 -> dig_p8/1
  I2C Read7/1 -> dig_p5/1
  I2C Read8/1 -> dig_p6/1

== system Copy_2_of_laod_arduino_2021/Misure Sensori/BMP_280/Subsystem ==
  T : Inport
  Cal_alt : Inport  Port=2
  T_01 : Inport  Port=3
  Constant : Constant  Value=15
  NotEqual : RelationalOperator  Operator=~=  OutDataTypeStr=boolean  RndMeth=Simplest
  Subsystem1 : Subsystem
  Switch : Switch  Criteria=u2 > Threshold
  Switch1 : Switch  Criteria=u2 > Threshold
  T_02 : Outport  VectorParamsAs1DForOutWhenUnconnected=off
  Cal_alt2 : Outport  Port=2  VectorParamsAs1DForOutWhenUnconnected=off
  wires:
  T_01/1 -> NotEqual/2, Switch1/1, Switch/3
  Switch1/1 -> T_02/1
  Switch/1 -> Switch1/3
  Constant/1 -> NotEqual/1
  Subsystem1/1(T_0) -> Switch/1, Switch/2
  NotEqual/1 -> Switch1/2
  Cal_alt/1 -> Cal_alt2/1, Subsystem1/Enable
  T/1 -> Subsystem1/1(T)

== system Copy_2_of_laod_arduino_2021/Misure Sensori/GPS_Venus/Subsystem1 ==
  h : Inport
  fix : Inport  Port=2
  Enable : EnablePort
  Constant : Constant
  Constant1 : Constant  Value=2
  Constant2 : Constant  Value=0
  Constant3 : Constant  Value=3
  Equal : RelationalOperator  Operator===  OutDataTypeStr=boolean  RndMeth=Simplest
  Equal1 : RelationalOperator  Operator===  OutDataTypeStr=boolean  RndMeth=Simplest
  Equal2 : RelationalOperator  Operator===  OutDataTypeStr=boolean  RndMeth=Simplest
  OR : Logic  Operator=OR  Inputs=3  IconShape=distinctive  AllPortsSameDT=off  OutDataTypeStr=boolean
  Switch : Switch  Criteria=u2 > Threshold
  h_to_subtract : Outport  VectorParamsAs1DForOutWhenUnconnected=off
  wires:
  Constant/1 -> Equal/2
  Equal/1 -> OR/1
  Constant1/1 -> Equal1/2
  Equal1/1 -> OR/2
  h/1 -> Switch/1
  OR/1 -> Switch/2
  Constant2/1 -> Switch/3
  Switch/1 -> h_to_subtract/1
  Equal2/1 -> OR/3
  Constant3/1 -> Equal2/2
  fix/1 -> Equal2/1, Equal1/1, Equal/1

== system Copy_2_of_laod_arduino_2021/Misure Sensori/GPS_Venus/Subsystem2 ==
  In1 : Inport
  Enable : EnablePort
  Create_message : MATLAB Function  TreatAsAtomicUnit=on
  Subsystem : Subsystem
  Misure_GPS : Outport  VectorParamsAs1DForOutWhenUnconnected=off
  mario : Outport  Port=2  VectorParamsAs1DForOutWhenUnconnected=off
  wires:
  In1/1 -> Create_message/1(byte_pack)
  Create_message/2(messaggio) -> Subsystem/1(In1)
  Create_message/1(status) -> Subsystem/Enable
  Subsystem/1(Outport) -> Misure_GPS/1
  Subsystem/2(mario) -> mario/1
